simulink model "Signal_Identification"  (R2016b)
settings: Solver=VariableStepAuto  StartTime=0.0  StopTime=3  MaxStep=1e-5  MinStep=1e-7
InitFcn:
  | ParameterSet
values from neighbouring files (symbols this model uses):
  Op_Time = 2    [ParameterSet.m]
libraries: simulink x1
settings Model: Creator=littlestar  LastModifiedBy=littlestar

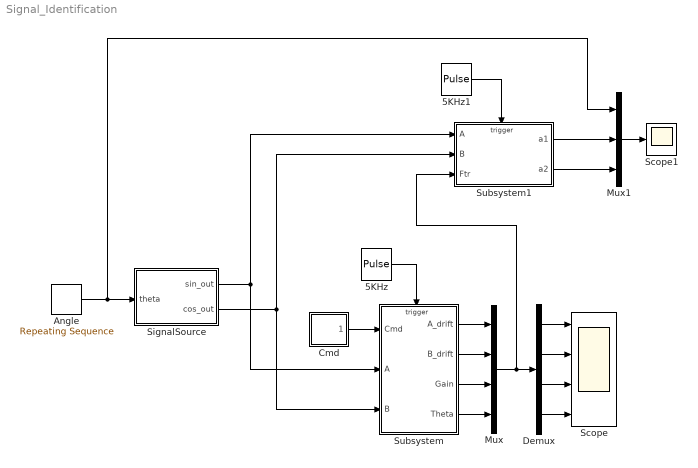
== system Signal_Identification ==
  5KHz : DiscretePulseGenerator  PulseType=Time based  Period=2e-4  PulseWidth=50
  5KHz1 : DiscretePulseGenerator  PulseType=Time based  Period=2e-4  PulseWidth=50
  Angle : simulink/Sources/Repeating Sequence  rep_seq_t=[0 0.01]  rep_seq_y=[0 2*pi]
  Cmd : Subsystem
      mask Display: disp('Cmd')
  Demux : Demux
  Mux : Mux
  Mux1 : Mux  Inputs=3
  Scope : Scope  NumInputPorts=4
  Scope1 : Scope
  SignalSource : MATLAB Function  TreatAsAtomicUnit=on
  Subsystem : Subsystem
      mask Display: disp('EllipseFitting')
  Subsystem1 : Subsystem
      mask Display: disp('AngleCalculate')
  wires:
  Angle/1 -> SignalSource/1(theta), Mux1/1
  SignalSource/1(sin_out) -> Subsystem/2(A), Subsystem1/1(A)
  SignalSource/2(cos_out) -> Subsystem1/2(B), Subsystem/3(B)
  5KHz/1 -> Subsystem/Trigger
  Cmd/1(Out1) -> Subsystem/1(Cmd)
  Subsystem/1(A_drift) -> Mux/1
  Subsystem/2(B_drift) -> Mux/2
  Subsystem/3(Gain) -> Mux/3
  Subsystem/4(Theta) -> Mux/4
  Mux/1 -> Demux/1, Subsystem1/3(Ftr)
  Demux/1 -> Scope/1
  Demux/2 -> Scope/2
  Demux/3 -> Scope/3
  Demux/4 -> Scope/4
  5KHz1/1 -> Subsystem1/Trigger
  Subsystem1/1(a1) -> Mux1/2
  Subsystem1/2(a2) -> Mux1/3
  Mux1/1 -> Scope1/1

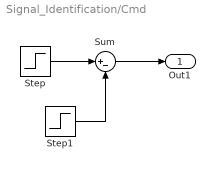
== system Signal_Identification/Cmd ==
  Step : Step  Time=0.2  SampleTime=0
  Step1 : Step  Time=0.2+Op_Time  SampleTime=0
  Sum : Sum  Inputs=|+-
  Out1 : Outport
  wires:
  Sum/1 -> Out1/1
  Step/1 -> Sum/1
  Step1/1 -> Sum/2

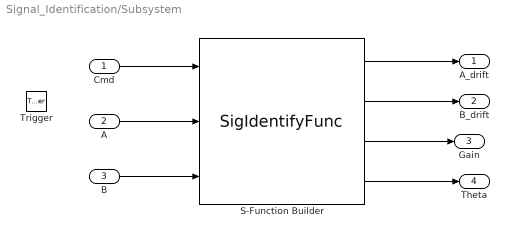
== system Signal_Identification/Subsystem ==
  Cmd : Inport
  A : Inport  Port=2
  B : Inport  Port=3
  Trigger : TriggerPort  VariantControl=Variant  PortDimensions=1
  S-Function Builder : S-Function  InitFcn=try, set_param(gcb,'FunctionName','SigIdentifyFunc'), end  FunctionName=SigIdentifyFunc  SFunctionModules=SigIdentifyFunc_wrapper  SFunctionDeploymentMode=off  EnableBusSupport=off  mask(S-Function Builder){}
      mask help: Simulink:masks:SFunctionBuilder_MD
      mask init:
      | val = [[.9  0.75 0.75 1 1 .9 .9 1]',[1 1 0.75 0.75 .9 .9 1 .9]'];try , sys = get_param(gcb,'SfunBuilderFcnName');if isempty(sys), sys = get_param(gcb,'FunctionName'); end,catch, sys = get_param(gcb,'FunctionName'); end
      settings: CopyFcn=set_param(gcbh,'LinkStatus','none')  PreSaveFcn=try, set_param(gcb,'FunctionName','SigIdentifyFunc'), end  OpenFcn=sfunctionwizard(gcbh)
      mask Display: plot(val(:,1),val(:,2)),disp(sys), port_label('input',1,'RunCmd'), port_label('input',2,'SignalA'), port_label('input',3,'SignalB'), port_label('output',1,'Sin_drift'), port_label('output',2,'Cos_drift'), port_label('output',3,'Gain'), port_label('output',4,'Theta')
  A_drift : Outport
  B_drift : Outport  Port=2
  Gain : Outport  Port=3
  Theta : Outport  Port=4
  wires:
  B/1 -> S-Function Builder/3
  Cmd/1 -> S-Function Builder/1
  S-Function Builder/1 -> A_drift/1
  A/1 -> S-Function Builder/2
  S-Function Builder/2 -> B_drift/1
  S-Function Builder/3 -> Gain/1
  S-Function Builder/4 -> Theta/1

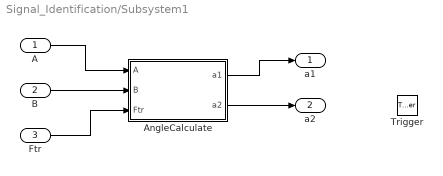
== system Signal_Identification/Subsystem1 ==
  A : Inport
  B : Inport  Port=2
  Ftr : Inport  Port=3
  Trigger : TriggerPort  VariantControl=Variant  PortDimensions=1
  AngleCalculate : MATLAB Function  TreatAsAtomicUnit=on
  a1 : Outport
  a2 : Outport  Port=2
  wires:
  A/1 -> AngleCalculate/1(A)
  B/1 -> AngleCalculate/2(B)
  AngleCalculate/2(a2) -> a2/1
  Ftr/1 -> AngleCalculate/3(Ftr)
  AngleCalculate/1(a1) -> a1/1

== matlab function Signal_Identification/Subsystem1/AngleCalculate ==
  data: A input; a1 output; B input; Ftr input; a2 output
function [a1,a2] = Calcu(A,B,Ftr)

%Calculate a1(without transforming)
if B == 0
    if A >= 0
        a1 = pi/2;
    else
        a1 = 3*pi/2;
    end
else
    if B < 0
        a1 = atan(A/B) + pi;
    else
        if A < 0
            a1 = atan(A/B) + 2*pi;
        else
            a1 = atan(A/B);
        end
    end
end

if a1 < 0
    a1 = a1 + 2*pi;
end

%Calculate a2
sintmp = sin(Ftr(4)/65536*2*pi);
costmp = cos(Ftr(4)/65536*2*pi);
A_tmp = A - Ftr(1);
B_tmp = (B - Ftr(2))*Ftr(3)/1024*costmp;

if B_tmp == 0
    if A_tmp >= 0
        a2 = pi/2;
    else
        a2 = -pi/2;
    end
else
    if B_tmp < 0
        a2 = atan((A_tmp/B_tmp)-(sintmp/costmp)) + pi;
    else
        if A_tmp < 0
            a2 = atan((A_tmp/B_tmp)-(sintmp/costmp)) + 2*pi;
        else
            a2 = atan((A_tmp/B_tmp)-(sintmp/costmp));
        end
    end
end

if a2 < 0
    a2 = a2 + 2*pi;
end

== matlab function Signal_Identification/SignalSource ==
  data: theta input; sin_out output; cos_out output
function [sin_out,cos_out] = Source(theta)

Gain_Err = 1.1;
Amp = 19859;  % (1V/3.3V)*65536
Drift1 = 300;
Drift2 = 500;
Theta_Err = 0.1745;

sin_out = Gain_Err * Amp * sin(theta + Theta_Err) + Drift1;
cos_out = Amp * cos(theta) + Drift2;
